simulink model "VRFT_IPC_dist"  (R2015a)
settings: Solver=ode3  StartTime=0.0  StopTime=TMax  FixedStep=DT  MaxStep=DT  RelTol=1e-3
values from neighbouring files (symbols this model uses):
  angleOpPoint = 8.672*pi/180    (= 0.151354952733)    [exe_VRFT_discreto.m]
  ControllerSampleTime = DTcontroller    [exe_VRFT_dataCollect.m]    (also in exe_VRFT_discreto.m = -1)
  denD = [ 1 -1]    [VRFTControllerLoad.m]
  denFilter = 1    [exe_VRFT_dataCollect.m]    (also in exe_VRFT_discreto.m)
  numD = [-0.02455 0.03899]    [VRFTControllerLoad.m]    (also in exe_VRFT_discreto.m = numD*GKaux(3))
  numFilter = 1    [exe_VRFT_dataCollect.m]    (also in exe_VRFT_discreto.m)
undefined symbols (not defined in the file or in its folder): avgtip_op, Avgyop, denD_IPC, DT, NDOF, numD_IPC, NumOuts, OutList, q_init, qdot_init, strmatch
settings Model: Creator=Vinicius  LastModifiedBy=mauri
settings DataIOCC: SignalLoggingSaveFormat=ModelDataLogs  SaveOutput=off  SaveTime=off  SignalLoggingName=sigsOut
settings OptimizationCC: ExpressionDepthLimit=2147483647
settings DebuggingCC: SaveWithParameterizedLinksMsg=none  UnderspecifiedInitializationDetection=Classic  MergeDetectMultiDrivingBlocksExec=none  SignalResolutionControl=TryResolveAllWithWarning  MultiTaskDSMMsg=warning  MultiTaskCondExecSysMsg=none  StateNameClashWarn=warning
settings HardwareCC: TargetLongLongMode=on  TargetIntDivRoundTo=Zero  TargetEndianess=LittleEndian  TargetHWDeviceType=MATLAB Host  ProdEqTarget=off
settings GRTTargetCC: CombineOutputUpdateFcns=off  GRTInterface=on

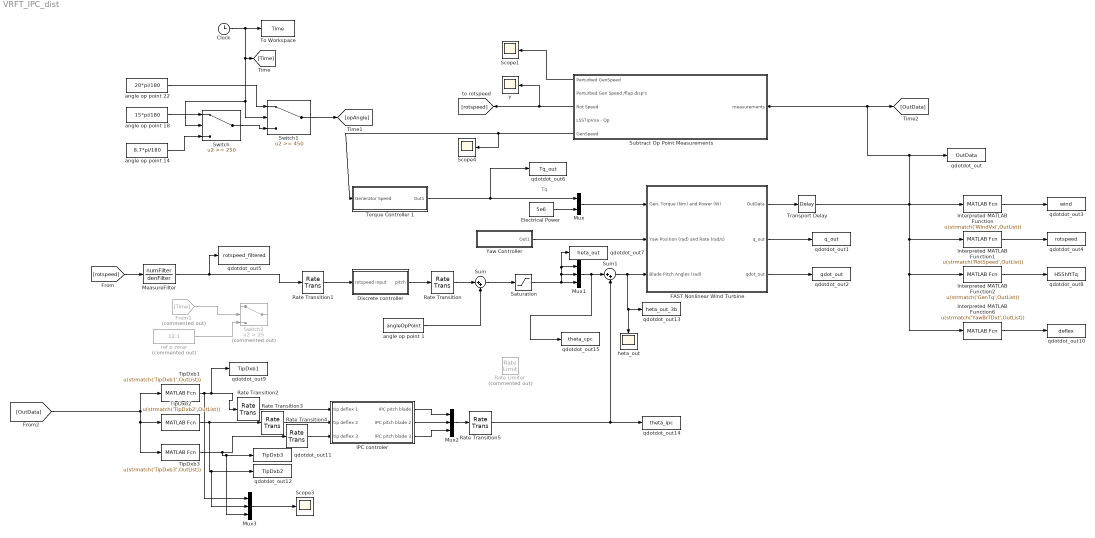
== system VRFT_IPC_dist ==
  note: Tq
  Clock : Clock
  Discrete controller : Subsystem
  Electrical Power : Constant  Value=5e6
  FAST Nonlinear Wind Turbine : Subsystem  mask(FAST Nonlinear Wind Turbine){}
      mask help: This block contains the FAST S-Function and blocks that integrate the DOF accelerations to get velocities and displacements.
      mask init:
      | clear FAST_SFunc
  From1 : From  Commented=on  GotoTag=Time
  IPC controler : Subsystem
  Interpreted MATLAB Function : MATLABFcn  MATLABFcn=u(strmatch('WindVxi',OutList))
  Interpreted MATLAB Function1 : MATLABFcn  MATLABFcn=u(strmatch('RotSpeed',OutList))
  Interpreted MATLAB Function2 : MATLABFcn  MATLABFcn=u(strmatch('GenTq',OutList))
  Interpreted MATLAB Function6 : MATLABFcn  MATLABFcn=u(strmatch('YawBrTDxt',OutList))
  MeasureFilter : TransferFcn  Numerator=numFilter  Denominator=denFilter
  Mux : Mux  Inputs=2
  Mux1 : Mux  Inputs=3
  Mux2 : Mux  Inputs=3
  Mux3 : Mux  Inputs=3
  Rate Limiter : RateLimiter  Commented=on  RisingSlewLimit=2*pi/180  FallingSlewLimit=-2*pi/180  SampleTimeMode=inherited
  Rate Transition{,1..5} (6 alike) : RateTransition
  Saturation : Saturate  UpperLimit=90*pi/180  LowerLimit=0
  Scope1 : Scope
      settings: TimeRange=79.99800000000001  YMin=-52  YMax=-30
  Scope3 : Scope
      settings: TimeRange=79.99800000000001  YMin=190  YMax=350  SaveName=ScopeData12
  Scope4 : Scope
      settings: TimeRange=79.99800000000001  YMin=190  YMax=350  SaveName=ScopeData2
  Subtract Op Point Measurements : Subsystem
  Sum : Sum  Inputs=|++
  Sum1 : Sum  Inputs=|++
  Switch : Switch  Threshold=250
  Switch1 : Switch  Threshold=450
  Switch2 : Switch  Commented=on  Criteria=u2 > Threshold  Threshold=25
  TipDxb1 : MATLABFcn  MATLABFcn=u(strmatch('TipDxb1',OutList))
  TipDxb2 : MATLABFcn  MATLABFcn=u(strmatch('TipDxb2',OutList))
  TipDxb3 : MATLABFcn  MATLABFcn=u(strmatch('TipDxb3',OutList))
  To Workspace : ToWorkspace  VariableName=Time  SampleTime=-1
  "Torque Controller 1 " : Subsystem
  Transport Delay : TransportDelay  DelayTime=1*DT
  Y : Scope
      settings: TimeRange=100  YMin=2.5  YMax=30  SaveName=ScopeData3
  Yaw Controller : Subsystem
  angle op point 1 : Constant  Value=angleOpPoint
  angle op point 14 : Constant  Value=8.7*pi/180
  "angle op point 18 " : Constant  Value=15*pi/180
  angle op point 22 : Constant  Value=20*pi/180
  heta_out : Scope
      settings: TimeRange=79.99800000000001  YMin=190  YMax=350  SaveName=ScopeData11
  qdotdot_out : ToWorkspace  VariableName=OutData  SampleTime=-1
  qdotdot_out1 : ToWorkspace  VariableName=q_out  SampleTime=-1
  qdotdot_out10 : ToWorkspace  VariableName=deflex  SampleTime=-1
  qdotdot_out11 : ToWorkspace  VariableName=TipDxb3  SampleTime=-1
  qdotdot_out12 : ToWorkspace  VariableName=TipDxb2  SampleTime=-1
  qdotdot_out13 : ToWorkspace  VariableName=heta_out_3b  SampleTime=-1
  qdotdot_out14 : ToWorkspace  VariableName=theta_ipc  SampleTime=-1
  qdotdot_out15 : ToWorkspace  VariableName=theta_cpc  SampleTime=-1
  qdotdot_out2 : ToWorkspace  VariableName=qdot_out  SampleTime=-1
  qdotdot_out3 : ToWorkspace  VariableName=wind  SampleTime=-1
  qdotdot_out4 : ToWorkspace  VariableName=rotspeed  SampleTime=-1
  qdotdot_out5 : ToWorkspace  VariableName=rotspeed_filtered  SampleTime=-1
  qdotdot_out6 : ToWorkspace  VariableName=Tq_out  SampleTime=-1
  qdotdot_out7 : ToWorkspace  VariableName=heta_out  SampleTime=-1
  qdotdot_out8 : ToWorkspace  VariableName=HSShftTq  SampleTime=-1
  qdotdot_out9 : ToWorkspace  VariableName=TipDxb1  SampleTime=-1
  ref p zerar : Constant  Commented=on  Value=12.1
  wires:
  Clock/1 -> Switch1/2, Switch/2, [Time], To Workspace/1
  FAST Nonlinear Wind Turbine/2(q_out) -> qdotdot_out1/1
  FAST Nonlinear Wind Turbine/3(qdot_out) -> qdotdot_out2/1
  Yaw Controller/1(Out1) -> FAST Nonlinear Wind Turbine/2(Yaw Position (rad) and Rate (rad/s))
  Electrical Power/1 -> Mux/2
  FAST Nonlinear Wind Turbine/1(OutData) -> Transport Delay/1
  Interpreted MATLAB Function/1 -> qdotdot_out3/1
  Interpreted MATLAB Function1/1 -> qdotdot_out4/1
  Interpreted MATLAB Function2/1 -> qdotdot_out8/1
  Mux/1 -> FAST Nonlinear Wind Turbine/1(Gen. Torque (Nm) and Power (W))
  "Torque Controller 1 "/1(Out1) -> qdotdot_out6/1, Mux/1
  Subtract Op Point Measurements/5(GenSpeed) -> Scope4/1, "Torque Controller 1 "/1(Generator Speed)
  Subtract Op Point Measurements/1(Perturbed GenSpeed) -> Scope1/1
  Subtract Op Point Measurements/3(Rot Speed) -> [rotspeed], Y/1
  Transport Delay/1 -> Interpreted MATLAB Function/1, qdotdot_out/1, Subtract Op Point Measurements/1(measurements), [OutData], Interpreted MATLAB Function6/1, Interpreted MATLAB Function2/1, Interpreted MATLAB Function1/1
  Interpreted MATLAB Function6/1 -> qdotdot_out10/1
  angle op point 14/1 -> Switch/3
  Switch/1 -> Switch1/3
  "angle op point 18 "/1 -> Switch/1
  angle op point 22/1 -> Switch1/1
  Switch1/1 -> [opAngle]
  Discrete controller/1("pitch ") -> Rate Transition/1
  Rate Transition1/1 -> Discrete controller/1(rotspeed input)
  angle op point 1/1 -> Sum/2
  Saturation/1 -> Mux1/2, Mux1/1, qdotdot_out7/1, Mux1/3
  [rotspeed] -> MeasureFilter/1
  From1/1 -> Switch2/2
  ref p zerar/1 -> Switch2/3
  Rate Transition/1 -> Sum/1
  Sum/1 -> Saturation/1
  MeasureFilter/1 -> Rate Transition1/1, qdotdot_out5/1
  TipDxb1/1 -> Mux3/1, qdotdot_out9/1, Rate Transition2/1
  TipDxb3/1 -> Rate Transition4/1, Mux3/3, qdotdot_out11/1
  TipDxb2/1 -> Rate Transition3/1, Mux3/2, qdotdot_out12/1
  Mux1/1 -> qdotdot_out15/1, Sum1/1
  Sum1/1 -> qdotdot_out13/1, heta_out/1, FAST Nonlinear Wind Turbine/3(Blade Pitch Angles (rad))
  IPC controler/2(IPC pitch blade 2) -> Mux2/2
  IPC controler/1("IPC pitch blade ") -> Mux2/1
  IPC controler/3(IPC pitch blade 3) -> Mux2/3
  Mux2/1 -> Rate Transition5/1
  Rate Transition2/1 -> IPC controler/1(tip deflex 1)
  Rate Transition3/1 -> IPC controler/2(tip deflex 2)
  Rate Transition4/1 -> IPC controler/3(tip deflex 3)
  Mux3/1 -> Scope3/1
  Rate Transition5/1 -> qdotdot_out14/1, Sum1/2
  [OutData] -> TipDxb3/1, TipDxb2/1, TipDxb1/1

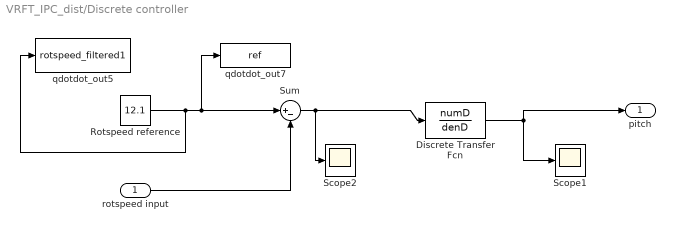
== system VRFT_IPC_dist/Discrete controller ==
  rotspeed input : Inport
  Discrete Transfer Fcn : DiscreteTransferFcn  Numerator=numD  Denominator=denD  SampleTime=ControllerSampleTime
  Rotspeed reference : Constant  Value=12.1
  Scope1 : Scope
      settings: YMin=-12000  YMax=1000
  Scope2 : Scope
      settings: SaveName=ScopeData5
  Sum : Sum  Inputs=|+-
  qdotdot_out5 : ToWorkspace  VariableName=rotspeed_filtered1  SampleTime=-1
  qdotdot_out7 : ToWorkspace  VariableName=ref  SampleTime=-1
  "pitch " : Outport
  wires:
  rotspeed input/1 -> Sum/2
  Rotspeed reference/1 -> qdotdot_out5/1, qdotdot_out7/1, Sum/1
  Sum/1 -> Discrete Transfer Fcn/1, Scope2/1
  Discrete Transfer Fcn/1 -> Scope1/1, "pitch "/1

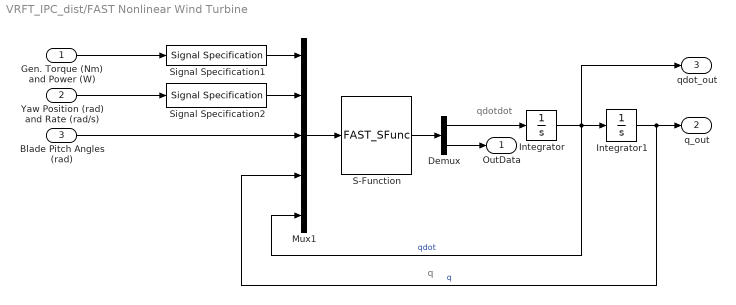
== system VRFT_IPC_dist/FAST Nonlinear Wind Turbine ==
  note: qdotdot
  note: q
  Gen. Torque (Nm) and Power (W) : Inport
  Yaw Position (rad) and Rate (rad/s) : Inport  Port=2
  Blade Pitch Angles (rad) : Inport  Port=3
  Demux : Demux  Outputs=[NDOF, NumOuts]
  Integrator : Integrator  InitialCondition=qdot_init
  Integrator1 : Integrator  InitialCondition=q_init
  Mux1 : Mux  Inputs=5
  S-Function : S-Function  FunctionName=FAST_SFunc
  Signal Specification1 : SignalSpecification  OutDataTypeStr=double  Dimensions=2
  Signal Specification2 : SignalSpecification  OutDataTypeStr=double  Dimensions=2
  OutData : Outport
  q_out : Outport  Port=2
  qdot_out : Outport  Port=3
  wires:
  Integrator/1 -> Mux1/5, qdot_out/1, Integrator1/1  "qdot"
  Gen. Torque (Nm) and Power (W)/1 -> Signal Specification1/1
  S-Function/1 -> Demux/1
  Demux/1 -> Integrator/1
  Demux/2 -> OutData/1
  Mux1/1 -> S-Function/1
  Blade Pitch Angles (rad)/1 -> Mux1/3
  Yaw Position (rad) and Rate (rad/s)/1 -> Signal Specification2/1
  Integrator1/1 -> q_out/1, Mux1/4  "q"
  Signal Specification1/1 -> Mux1/1
  Signal Specification2/1 -> Mux1/2

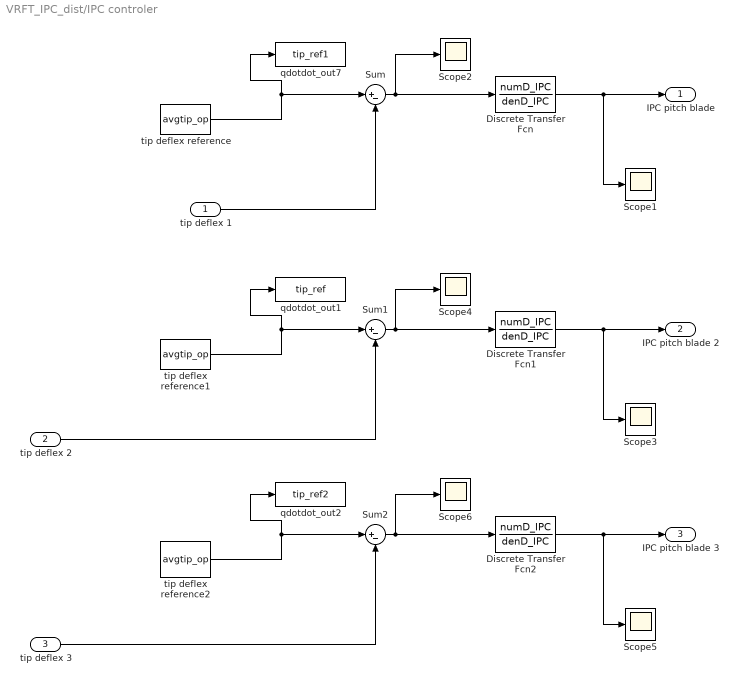
== system VRFT_IPC_dist/IPC controler ==
  tip deflex 1 : Inport
  tip deflex 2 : Inport  Port=2
  tip deflex 3 : Inport  Port=3
  Discrete Transfer Fcn : DiscreteTransferFcn  Numerator=numD_IPC  Denominator=denD_IPC  SampleTime=ControllerSampleTime
  Discrete Transfer Fcn1 : DiscreteTransferFcn  Numerator=numD_IPC  Denominator=denD_IPC  SampleTime=ControllerSampleTime
  Discrete Transfer Fcn2 : DiscreteTransferFcn  Numerator=numD_IPC  Denominator=denD_IPC  SampleTime=ControllerSampleTime
  Scope{1..6} (6 alike) : Scope
      Scope1 settings: YMin=-12000  YMax=1000  SaveName=ScopeData4
      Scope2 settings: SaveName=ScopeData6
      Scope3 settings: YMin=-12000  YMax=1000  SaveName=ScopeData7
      Scope4 settings: SaveName=ScopeData8
      Scope5 settings: YMin=-12000  YMax=1000  SaveName=ScopeData9
      Scope6 settings: SaveName=ScopeData10
  Sum : Sum  Inputs=|+-
  Sum1 : Sum  Inputs=|+-
  Sum2 : Sum  Inputs=|+-
  qdotdot_out1 : ToWorkspace  VariableName=tip_ref  SampleTime=-1
  qdotdot_out2 : ToWorkspace  VariableName=tip_ref2  SampleTime=-1
  qdotdot_out7 : ToWorkspace  VariableName=tip_ref1  SampleTime=-1
  tip deflex reference : Constant  Value=avgtip_op
  tip deflex reference1 : Constant  Value=avgtip_op
  tip deflex reference2 : Constant  Value=avgtip_op
  "IPC pitch blade " : Outport
  IPC pitch blade 2 : Outport  Port=2
  IPC pitch blade 3 : Outport  Port=3
  wires:
  Discrete Transfer Fcn/1 -> Scope1/1, "IPC pitch blade "/1
  tip deflex 1/1 -> Sum/2
  tip deflex reference/1 -> qdotdot_out7/1, Sum/1
  Sum/1 -> Scope2/1, Discrete Transfer Fcn/1
  Discrete Transfer Fcn1/1 -> IPC pitch blade 2/1, Scope3/1
  tip deflex 2/1 -> Sum1/2
  tip deflex reference1/1 -> qdotdot_out1/1, Sum1/1
  Sum1/1 -> Scope4/1, Discrete Transfer Fcn1/1
  Discrete Transfer Fcn2/1 -> IPC pitch blade 3/1, Scope5/1
  tip deflex 3/1 -> Sum2/2
  tip deflex reference2/1 -> qdotdot_out2/1, Sum2/1
  Sum2/1 -> Scope6/1, Discrete Transfer Fcn2/1

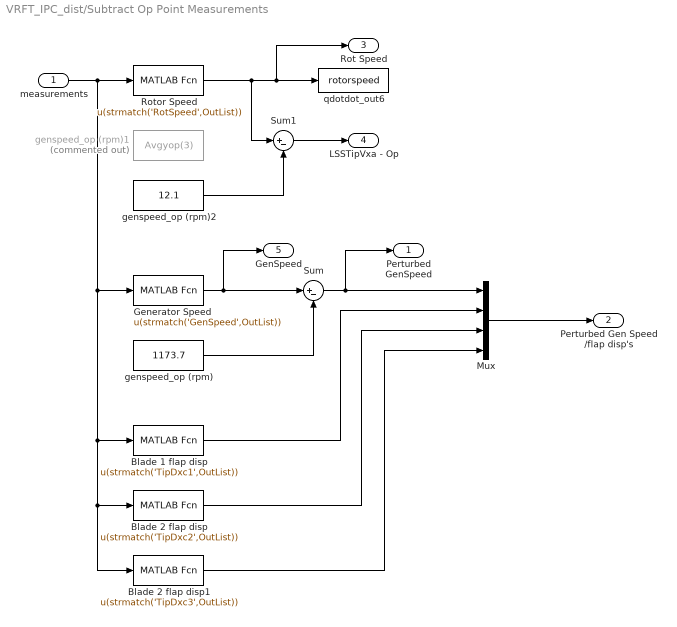
== system VRFT_IPC_dist/Subtract Op Point Measurements ==
  measurements : Inport
  Blade 1 flap disp : MATLABFcn  MATLABFcn=u(strmatch('TipDxc1',OutList))
  Blade 2 flap disp : MATLABFcn  MATLABFcn=u(strmatch('TipDxc2',OutList))
  Blade 2 flap disp1 : MATLABFcn  MATLABFcn=u(strmatch('TipDxc3',OutList))
  Generator Speed : MATLABFcn  MATLABFcn=u(strmatch('GenSpeed',OutList))
  Mux : Mux
  Rotor Speed : MATLABFcn  MATLABFcn=u(strmatch('RotSpeed',OutList))
  Sum : Sum  Inputs=|+-
  Sum1 : Sum  Inputs=|+-
  genspeed_op (rpm) : Constant  Value=1173.7
  genspeed_op (rpm)1 : Constant  Commented=on  Value=Avgyop(3)
  genspeed_op (rpm)2 : Constant  Value=12.1
  qdotdot_out6 : ToWorkspace  VariableName=rotorspeed  SampleTime=-1
  Perturbed GenSpeed : Outport
  Perturbed Gen Speed /flap disp's : Outport  Port=2
  Rot Speed : Outport  Port=3
  LSSTipVxa - Op : Outport  Port=4
  GenSpeed : Outport  Port=5
  wires:
  Rotor Speed/1 -> Sum1/1, Rot Speed/1, qdotdot_out6/1
  Sum/1 -> Perturbed GenSpeed/1, Mux/1
  Blade 1 flap disp/1 -> Mux/2
  Blade 2 flap disp/1 -> Mux/3
  Blade 2 flap disp1/1 -> Mux/4
  measurements/1 -> Blade 2 flap disp/1, Blade 2 flap disp1/1, Blade 1 flap disp/1, Generator Speed/1, Rotor Speed/1
  genspeed_op (rpm)/1 -> Sum/2
  Generator Speed/1 -> GenSpeed/1, Sum/1
  Mux/1 -> Perturbed Gen Speed /flap disp's/1
  Sum1/1 -> LSSTipVxa - Op/1
  genspeed_op (rpm)2/1 -> Sum1/2

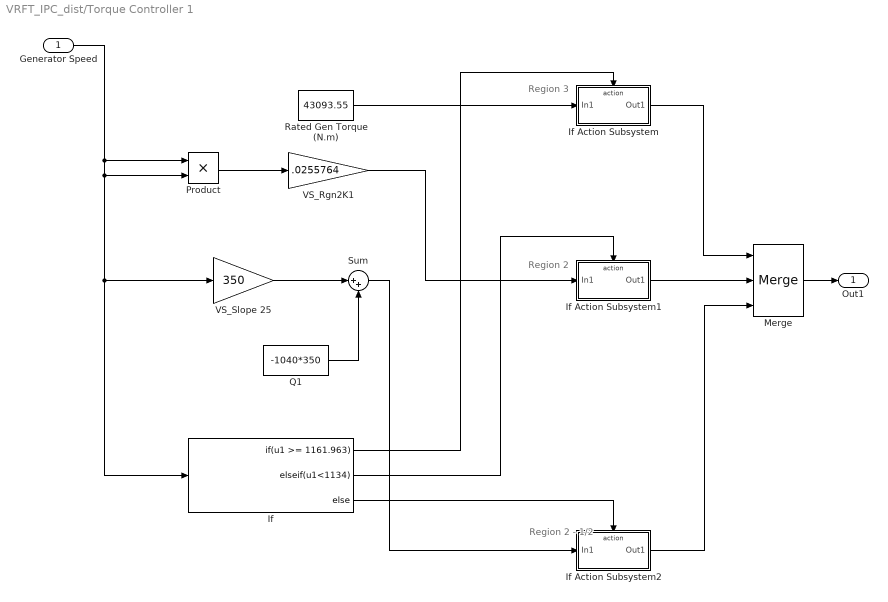
== system VRFT_IPC_dist/Torque Controller 1  ==
  note: Region 2 - 1/2
  note: Region 2
  note: Region 3
  Generator Speed : Inport
  If : If  IfExpression=u1 >= 1161.963  ElseIfExpressions=u1<1134
  If Action Subsystem : Subsystem  TreatAsAtomicUnit=on
  If Action Subsystem1 : Subsystem  TreatAsAtomicUnit=on
  If Action Subsystem2 : Subsystem  TreatAsAtomicUnit=on
  Merge : Merge  Inputs=3
  Product : Product  RndMeth=Zero
  Q1 : Constant  Value=-1040*350
  Rated Gen Torque (N.m) : Constant  Value=43093.55
  Sum : Sum  Inputs=|++
  VS_Rgn2K1 : Gain  Gain=.0255764
  VS_Slope 25 : Gain  Gain=350
  Out1 : Outport
  wires:
  Rated Gen Torque (N.m)/1 -> If Action Subsystem/1(In1)
  If/1 -> If Action Subsystem/Action
  If/2 -> If Action Subsystem1/Action
  If/3 -> If Action Subsystem2/Action
  If Action Subsystem2/1(Out1) -> Merge/3
  If Action Subsystem1/1(Out1) -> Merge/2
  If Action Subsystem/1(Out1) -> Merge/1
  Merge/1 -> Out1/1
  Generator Speed/1 -> Product/1, Product/2, VS_Slope 25/1, If/1
  Product/1 -> VS_Rgn2K1/1
  Q1/1 -> Sum/2
  VS_Slope 25/1 -> Sum/1
  Sum/1 -> If Action Subsystem2/1(In1)
  VS_Rgn2K1/1 -> If Action Subsystem1/1(In1)

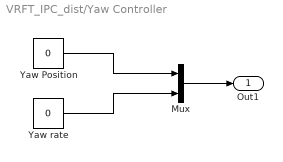
== system VRFT_IPC_dist/Yaw Controller ==
  Mux : Mux  Inputs=2
  Yaw Position : Constant  Value=0
  Yaw rate : Constant  Value=0
  Out1 : Outport
  wires:
  Mux/1 -> Out1/1
  Yaw Position/1 -> Mux/1
  Yaw rate/1 -> Mux/2

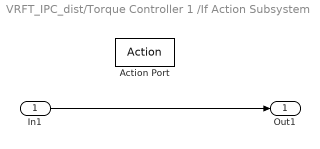
== system VRFT_IPC_dist/Torque Controller 1 /If Action Subsystem ==
  In1 : Inport
  Action Port : ActionPort  ActionType=then
  Out1 : Outport
  wires:
  In1/1 -> Out1/1

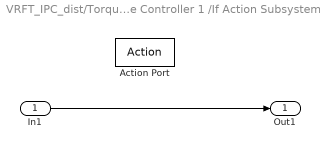
== system VRFT_IPC_dist/Torque Controller 1 /If Action Subsystem1 ==
  In1 : Inport
  Action Port : ActionPort  ActionType=elseif
  Out1 : Outport
  wires:
  In1/1 -> Out1/1

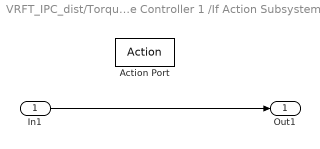
== system VRFT_IPC_dist/Torque Controller 1 /If Action Subsystem2 ==
  In1 : Inport
  Action Port : ActionPort  ActionType=else
  Out1 : Outport
  wires:
  In1/1 -> Out1/1
